simulink model "Modulation_DSBSC_AWGN_SNR"  (R2023a)
settings: Solver=VariableStepAuto  StartTime=0.0  StopTime=1  RelTol=1e-3
libraries: commchan3 x1, dspfdesign x1
settings Model: Creator=Pedro  LastModifiedBy=Pedro

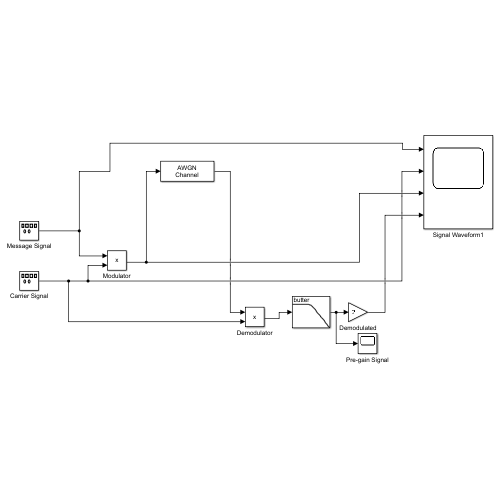
[thumbnail: Simulink's stored preview of the top-level diagram]
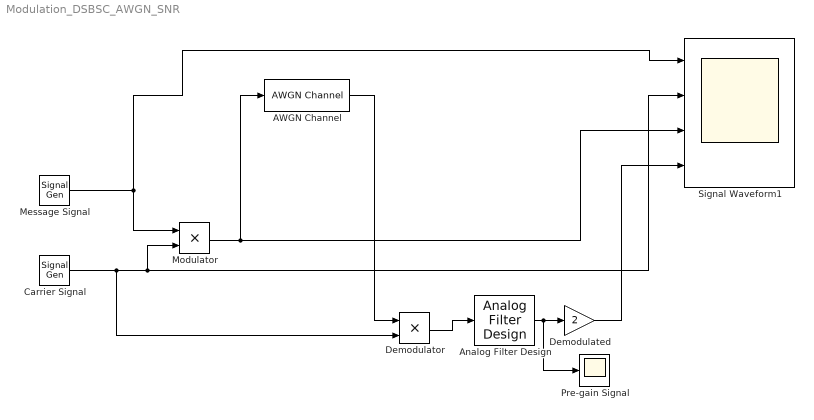
== system Modulation_DSBSC_AWGN_SNR ==
  AWGN Channel : commchan3/AWGN Channel  LegacyMode=off  NoiseMethod="Signal to noise ratio  (SNR)"  noiseMode="Signal to noise ratio  (SNR)"  EbNo=10  EsNo=10  SNR=23  BitsPerSymbol=1  SignalPower=1  SamplesPerSymbol=1  SymbolPeriod=1  VarianceSource=Parameter  Variance=1  RandomStream=Global stream  Seed=67  SimulateUsing=Code generation
  Analog Filter Design : dspfdesign/Analog Filter Design  method=Butterworth  filttype=Lowpass  N=4  Wlo=2*pi*40  Whi=80  Rp=2  Rs=40
  Carrier Signal : SignalGenerator  Frequency=110
  Demodulated : Gain  Gain=2
  Demodulator : Product
  Message Signal : SignalGenerator  Frequency=20
  Modulator : Product
  Pre-gain Signal : Scope
  Signal Waveform1 : Scope  NumInputPorts=4
  wires:
  Modulator/1 -> Signal Waveform1/3, AWGN Channel/1
  Message Signal/1 -> Signal Waveform1/1, Modulator/1
  Carrier Signal/1 -> Demodulator/2, Signal Waveform1/2, Modulator/2
  AWGN Channel/1 -> Demodulator/1
  Demodulator/1 -> Analog Filter Design/1
  Analog Filter Design/1 -> Pre-gain Signal/1, Demodulated/1
  Demodulated/1 -> Signal Waveform1/4
